simulink model "HighwayLaneFollowingTestBench"  (R2022a)
settings: Solver=ode23tb  StartTime=0.0  StopTime=scenario.StopTime  RelTol=1e-3
PostLoadFcn:
  | helperSLHighwayLaneFollowingSetup
values from neighbouring files (symbols this model uses):
  vehSim3D = repmat(     struct(         'Length', 0,         'RearOverhang', 0,         'InitialPos',[0 0 0],         'InitialRot',[0 0 0]),     numVehicles,1)    [helperSLHighwayLaneFollowingSetup.m]
undefined symbols (not defined in the file or in its folder): assessment, Ts, v_set
libraries: drivingscenarioandsensors x8, sim3dautolib x6, simulink x4, sim3dcameralib x1, sim3dprobsensorlib x1, sim3dlib x1, dspvision x1
CloseFcn:
  | helperSLHighwayLaneFollowingCleanUp
settings Model: SILPILSystemUnderTest=refmodels  Creator=The MathWorks, Inc.  LastModifiedBy=The MathWorks, Inc.
settings SolverCC: AlgebraicLoopSolver=TrustRegion  MaxZcPerStep=1
settings DataIOCC: SaveOutput=off  SaveTime=off  ReturnWorkspaceOutputs=off
settings DebuggingCC: ParameterPrecisionLossMsg=none  UnconnectedInputMsg=warning  UnconnectedOutputMsg=warning  UnconnectedLineMsg=warning  PregeneratedLibrarySubsystemCodeDiagnostic=none  SFMachineParentedDataDiag=warning  ArithmeticOperatorsInVariantConditions=warning
settings HardwareCC: ProdLongLongMode=on
settings SFSimCC: SimUseLocalCustomCode=off
settings RTWCC: RTWUseLocalCustomCode=off  DLArmComputeVersion=19.05
settings GRTTargetCC: RTWCAPISignals=on
settings ConfigComp: CovScope=ReferencedModels  CovIncludeTopModel=off

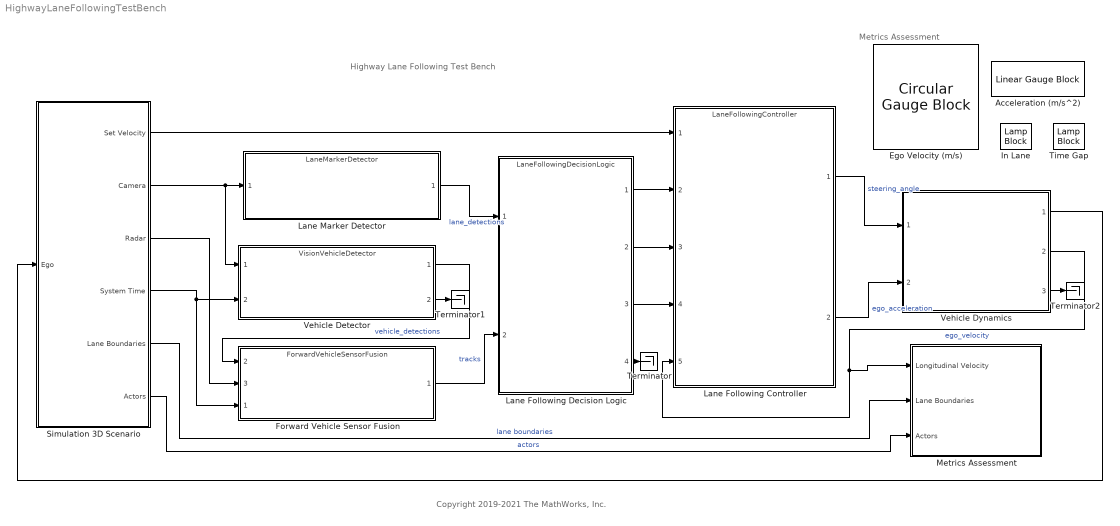
== system HighwayLaneFollowingTestBench ==
  note: Highway Lane Following Test Bench
  note: Metrics Assessment
  note: Copyright 2019-2021 The MathWorks, Inc.
  Acceleration (m/s^2) : LinearGaugeBlock  LabelPosition=Hide  ScaleMin=-6  ScaleMax=6
  Ego Velocity (m/s) : CircularGaugeBlock  LabelPosition=Hide  ScaleMax=50
  Forward Vehicle Sensor Fusion : ModelReference  ModelNameDialog=ForwardVehicleSensorFusion.slx  SimulationMode=Normal  CodeInterface=Top model  ModelReferenceVersion=5.7
      settings: PortSchema="{\"entries\":[{\"content\":{\"sides\":[{\"content\":{\"connectorIds\":[\"In2\",\"In3\",\"In1\"]},\"type\":\"ConnectorPlacement.EquallySpacedRectSide\",\"uuid\":\"7686684e-3ce8-49a8-9c28-78afc562c6cd\"},{\"content\":{\"connectorIds\":[\"Out1\"],\"side\":\"RIGHT\"},\"type\":\"ConnectorPlacement.EquallySpacedRectSide\",\"uuid\":\"c415bca7-2ba8-48d1-9f28-43832dd5ba4e\"},{\"content\":{\"connectorIds\":[],\"side\":\"TOP\"},\"type\":\"ConnectorPlacement.EquallySpacedRectSide\",\"uuid\":\"f22886ed-f0b4-4628-af34-640797a1171b\"}]},\"type\":\"ConnectorPlacement.EquallySpacedConnector\",\"uuid\":\"6b238f4e-3dd4-4f3d-8d3a-ef3e86789fb5\"}],\"packageUris\":[\"http://schema.mathworks.com/mf0/Connector/R2020b\"],\"version\":\"1.0\"}"
  In Lane : LampBlock  LabelPosition=Hide
  Lane Following Controller : ModelReference  ModelNameDialog=LaneFollowingController  SimulationMode=Normal  CodeInterface=Top model  ModelReferenceVersion=5.0
  Lane Following Decision Logic : ModelReference  ModelNameDialog=LaneFollowingDecisionLogic.slx  SimulationMode=Normal  CodeInterface=Top model  ModelReferenceVersion=4.0
  Lane Marker Detector : ModelReference  ModelNameDialog=LaneMarkerDetector.slx  SimulationMode=Normal  CodeInterface=Top model  ModelReferenceVersion=3.0
  Metrics Assessment : Subsystem
  Simulation 3D Scenario : Subsystem  VariantControl=1
  Terminator : Terminator
  Terminator1 : Terminator
  Terminator2 : Terminator
  Time Gap : LampBlock  LabelPosition=Hide
  Vehicle Detector : ModelReference  ModelNameDialog=VisionVehicleDetector.slx  SimulationMode=Normal  CodeInterface=Top model  ModelReferenceVersion=4.0
  Vehicle Dynamics : Subsystem  VariantControl=Variant2  ReferencedSubsystem=BicycleWithForceInput
  wires:
  Vehicle Dynamics/2 -> Lane Following Controller/5, Metrics Assessment/1(Longitudinal Velocity)  "ego_velocity"
  Vehicle Dynamics/1 -> Simulation 3D Scenario/1(Ego)
  Simulation 3D Scenario/6(Actors) -> Metrics Assessment/3(Actors)  "actors"
  Lane Following Controller/1 -> Vehicle Dynamics/1  "steering_angle"
  Lane Following Controller/2 -> Vehicle Dynamics/2  "ego_acceleration"
  Forward Vehicle Sensor Fusion/1 -> Lane Following Decision Logic/2  "tracks"
  Simulation 3D Scenario/5(Lane Boundaries) -> Metrics Assessment/2(Lane Boundaries)  "lane boundaries"
  Simulation 3D Scenario/3(Radar) -> Forward Vehicle Sensor Fusion/3
  Lane Marker Detector/1 -> Lane Following Decision Logic/1  "lane_detections"
  Simulation 3D Scenario/1(Set Velocity) -> Lane Following Controller/1
  Simulation 3D Scenario/4(System Time) -> Forward Vehicle Sensor Fusion/1, Vehicle Detector/2
  Simulation 3D Scenario/2(Camera) -> Vehicle Detector/1, Lane Marker Detector/1
  Lane Following Decision Logic/1 -> Lane Following Controller/2
  Lane Following Decision Logic/2 -> Lane Following Controller/3
  Lane Following Decision Logic/3 -> Lane Following Controller/4
  Vehicle Detector/2 -> Terminator1/1
  Vehicle Detector/1 -> Forward Vehicle Sensor Fusion/2  "vehicle_detections"
  Lane Following Decision Logic/4 -> Terminator/1
  Vehicle Dynamics/3 -> Terminator2/1

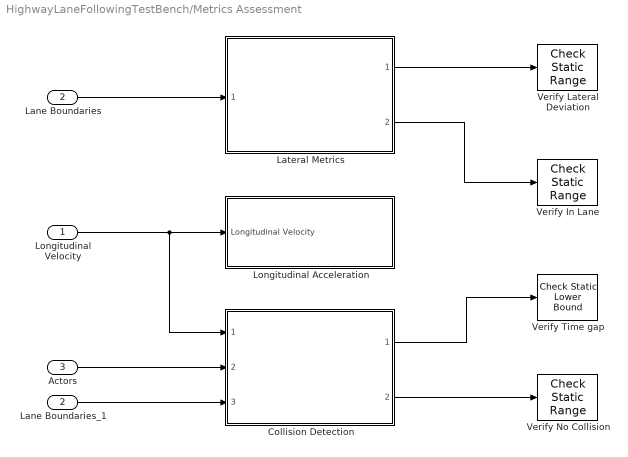
== system HighwayLaneFollowingTestBench/Metrics Assessment ==
  Longitudinal Velocity : Inport
  Lane Boundaries : Inport  Port=2
  Actors : Inport  Port=3
  Collision Detection : Subsystem  ReferencedSubsystem=CollisionDetection
  Lane Boundaries_1 : InportShadow  Port=2
  Lateral Metrics : Subsystem  ReferencedSubsystem=LateralMetrics
  Longitudinal Acceleration : Subsystem
  Verify In Lane : simulink/Model Verification/Check  Static Range  Description=1 <= u <= 1  max=1  max_included=on  min=1  min_included=on  enabled=on  stopWhenAssertionFail=on  export=off  icon=graphic
      settings: SourceProductBaseCode=SL
  Verify Lateral Deviation : simulink/Model Verification/Check  Static Range  Description=-assessment.LateralDeviationMax <= u <= assessment.LateralDeviationMax  max=assessment.LateralDeviationMax  max_included=on  min=-assessment.LateralDeviationMax  min_included=on  enabled=on  stopWhenAssertionFail=on  export=off  icon=graphic
      settings: SourceProductBaseCode=SL
      settings: AttributesFormatString=|
      | ---------------------------------------
      | max = %<max>
      | min = %<min>
  Verify No Collision : simulink/Model Verification/Check  Static Range  Description=0 <= u <= 0  max=0  max_included=on  min=0  min_included=on  enabled=on  stopWhenAssertionFail=on  export=off  icon=graphic
      settings: SourceProductBaseCode=SL
  Verify Time gap : simulink/Model Verification/Check Static  Lower Bound  Description=assessment.TimeGap <= u  min=assessment.TimeGap  min_included=on  enabled=on  stopWhenAssertionFail=on  export=off  icon=graphic
      settings: AttributesFormatString=|
      | ---------------------------------------
      | min = %<min>
  wires:
  Lane Boundaries/1 -> Lateral Metrics/1
  Collision Detection/1 -> Verify Time gap/1
  Lateral Metrics/1 -> Verify Lateral Deviation/1
  Collision Detection/2 -> Verify No Collision/1
  Longitudinal Velocity/1 -> Collision Detection/1, Longitudinal Acceleration/1(Longitudinal Velocity)
  Actors/1 -> Collision Detection/2
  Lateral Metrics/2 -> Verify In Lane/1
  Lane Boundaries_1/1 -> Collision Detection/3

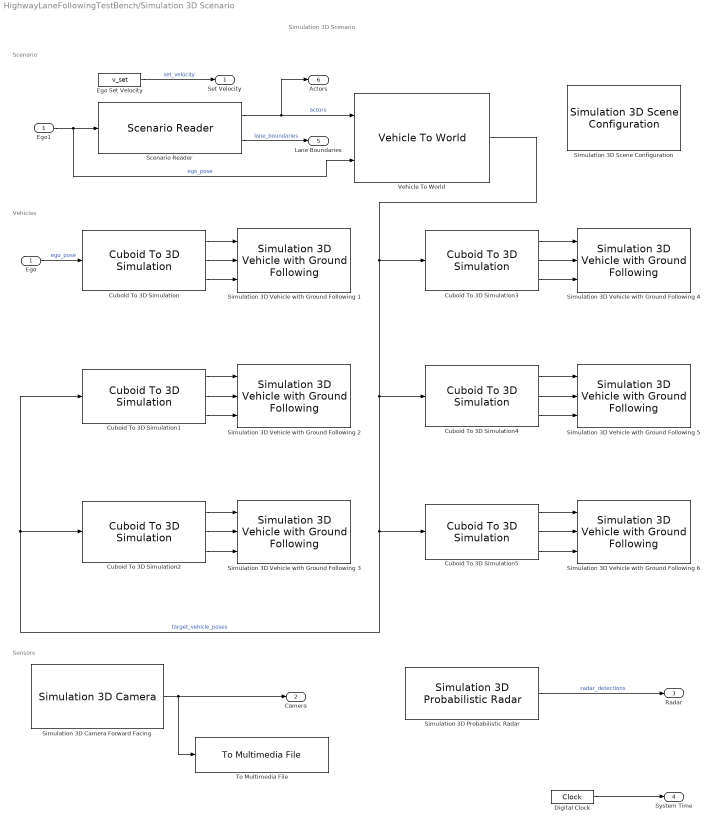
== system HighwayLaneFollowingTestBench/Simulation 3D Scenario ==
  note: Scenario
  note: Vehicles
  note: Simulation 3D Scenario
  note: Sensors
  Ego : Inport
  Cuboid To 3D Simulation : drivingscenarioandsensors/Cuboid To 3D Simulation  SpecifyActorID=off  ActorIDToConvert=1  SimulateUsing=Interpreted execution
      settings: SourceProductBaseCode=DR
  Cuboid To 3D Simulation1 : drivingscenarioandsensors/Cuboid To 3D Simulation  SpecifyActorID=on  ActorIDToConvert=2  SimulateUsing=Interpreted execution
      settings: SourceProductBaseCode=DR
  Cuboid To 3D Simulation2 : drivingscenarioandsensors/Cuboid To 3D Simulation  SpecifyActorID=on  ActorIDToConvert=3  SimulateUsing=Interpreted execution
      settings: SourceProductBaseCode=DR
  Cuboid To 3D Simulation3 : drivingscenarioandsensors/Cuboid To 3D Simulation  SpecifyActorID=on  ActorIDToConvert=4  SimulateUsing=Interpreted execution
      settings: SourceProductBaseCode=DR
  Cuboid To 3D Simulation4 : drivingscenarioandsensors/Cuboid To 3D Simulation  SpecifyActorID=on  ActorIDToConvert=5  SimulateUsing=Interpreted execution
      settings: SourceProductBaseCode=DR
  Cuboid To 3D Simulation5 : drivingscenarioandsensors/Cuboid To 3D Simulation  SpecifyActorID=on  ActorIDToConvert=6  SimulateUsing=Interpreted execution
      settings: SourceProductBaseCode=DR
  Digital Clock : DigitalClock  SampleTime=Ts
  Ego Set Velocity : Constant  Value=v_set  SampleTime=Ts
  Ego1 : InportShadow
  Scenario Reader : drivingscenarioandsensors/Scenario Reader  ScenarioSource=From workspace  ScenarioFileName=dblLaneChangeDrivingScenario.mat  ScenarioVariableName=scenario  OutputCoordinateSystem=Vehicle coordinates  EgoVehicleSource=Input port  EgoVehicleActorID=1  OrientVehiclesOnRoad=off  OutputEgoVehiclePose=off  OutputEgoVehicleState=off  SampleTime=0.1  LaneBoundaryOutput=Ego vehicle lane boundaries  LaneBoundaryDistance=0:0.5:70  LaneBoundaryLocation=Center of lane markings  BusNameSource=Auto  BusName=BusActors  BusNumActorsSource=Scenario  BusNumActors=100  BusName2Source=Auto  BusName2=BusLaneBoundaries  BusNumLaneBoundariesSource=Scenario  BusNumLaneBoundaries=10  BusName3Source=Auto  BusName3=BusEgoActor  BusName4Source=Auto  BusName4=BusEgoState  ShowCoordinateLabels=on  SimulateUsing=Interpreted execution
  Simulation 3D Camera Forward Facing : sim3dcameralib/Simulation 3D Camera  Priority=1  sensorTag=Sim3dSensor1  sensorId=1  sensorName=Sim3dSensor1  vehTagList={'Scene Origin';'SimulinkVehicle1';'SimulinkVehicle4';'SimulinkVehicle5';'SimulinkVehicle6';'vehSim3D(2).InitialRot';'vehSim3D(3).InitialRot'}  vehTag=SimulinkVehicle1  mountLoc=Origin  offsetFlag=on  tmountOffset=camera.PositionSim3d  extTmount=off  rmountOffset=camera.Rotation  extRmount=off  FocalLength=camera.FocalLength  OpticalCenter=camera.PrincipalPoint  ImageSize=camera.ImageSize  RadialDistortion=[0, 0]  TangentialDistortion=[0, 0]  SensorSkew=0  DepthOutportEnabled=off  SemanticOutportEnabled=off  TransformOutportEnabled=off  SampleTime=-1  mountPoint=[0.57 0 1.2]  mountOrientation=[0 0 0]  aMode=3  ID=1
      settings: SourceProductBaseCode=VE,AE,DR,UV,VE
      settings: AttributesFormatString=|
      | -------------------------------------
      | ImageSize = %<ImageSize>
      | OpticalCenter = %<OpticalCenter>
      | FocalLength = %<FocalLength>
      | RadialDistortion = %<RadialDistortion>
      | mountLoc = %<mountLoc>
      | tmountOffset = %<tmountOffset>
      | rmountOffset = %<rmountOffset>
      | Priority = %<Priority>
  Simulation 3D Probabilistic Radar : sim3dprobsensorlib/Simulation 3D Probabilistic Radar  Priority=1  sensorTag=Sim3dSensor2  sensorId=2  sensorName=Sim3dSensor2  vehTagList={'Scene Origin';'SimulinkVehicle1';'SimulinkVehicle4';'SimulinkVehicle5';'SimulinkVehicle6';'vehSim3D(2).InitialRot';'vehSim3D(3).InitialRot'}  vehTag=SimulinkVehicle1  mountLoc=Origin  offsetFlag=on  tmountOffset=radar.PositionSim3d  rmountOffset=radar.Rotation  AzimuthResolution=0.8  ElevationResolution=8  RangeResolution=1  RangeRateResolution=1  AzimuthBiasFraction=0.1  ElevationBiasFraction=0.1  RangeBiasFraction=0.05  RangeRateBiasFraction=0.05  FieldOfView=radar.FieldOfView  DetectionRange=radar.DetectionRanges  RangeRateLimits=[ -100, 100 ]  DetectionProbability=0.9  FalseAlarmRate=1e-6  ReferenceRange=150  ReferenceRCS=0  HasElevation=off  HasRangeRate=on  HasNoise=off  HasFalseAlarms=off  InitialSeedSource=Repeatable  InitialSeed=0  MaxNumDetections=50  DetectionCoordinates=Sensor spherical  SpecifyOutputBusName=off  BusName=BusSimulation3DRadarTruthSensor  SampleTime=-1  mountPoint=[2.424 0 0.8]  mountOrientation=[0 0 0]  aMode=3  ID=2
      settings: SourceProductBaseCode=VE,AE,DR,UV,VE
      settings: AttributesFormatString=|
      | -------------------------------------
      | FieldOfView = %<FieldOfView>
      | AzimuthResolution = %<AzimuthResolution>
      | DetectionCoordinates = %<DetectionCoordinates>
      | mountLoc = %<mountLoc>
      | tmountOffset = %<tmountOffset>
      | rmountOffset = %<rmountOffset>
      | Priority = %<Priority>
  Simulation 3D Scene Configuration : sim3dlib/Simulation 3D Scene Configuration  Priority=0  ProjectFormat=Default Scenes  SceneDesc=Curved road  ProjectName=/mathworks/devel/bat/BR2022ad/build/matlab/toolbox/shared/sim3d_projects/automotive_project/UE4/LinuxNoEditor/AutoVrtlEnv.sh  ScenePath=/Game/Maps/HwStrght  vehTagList={'Scene Origin';'SimulinkVehicle1';'SimulinkVehicle4';'SimulinkVehicle5';'SimulinkVehicle6';'vehSim3D(2).InitialRot';'vehSim3D(3).InitialRot'}  vehTag=SimulinkVehicle1  OpVisEn=off  Ts=0.1  EnableWindow=on  EnableRemoteAccess=off  EnableWeather=off  SunAltitude=40.0  SunAzimuth=90  clouds=10  wind=1  fog=0  rain=0  sensorTag=MainCamera1  sensorId=1  sensorName=MainCamera1  mountLoc=Origin  offsetFlag=off  tmountOffset=[0, 0, 0]  rmountOffset=[0, 0, 0]  HorizontalResolution=1280  VerticalResolution=720  HorizontalFOV=60  mountPoint=[0 0 0]  mountOrientation=[0 0 0]  aMode=3  ID=1
      settings: SourceProductBaseCode=VE,AE,DR,UV,VE
      settings: AttributesFormatString=|
      | -------------------------------------
      | SceneName = %<SceneDesc>
      | Priority = %<Priority>
  Simulation 3D Vehicle with Ground Following 1 : sim3dautolib/Simulation 3D Vehicle with Ground Following  Priority=-1  PassVehMesh=Sedan  MeshPath=/MathWorksSimulation/Vehicles/Muscle/Meshes/SK_MuscleCar.SK_MuscleCar  TrackWidth=1.9  WheelBase=3  WheelRadius=0.35  VehColor=Blue  InitialPos=vehSim3D(1).InitialPos  InitialRot=vehSim3D(1).InitialRot  ActorName=SimulinkVehicle1  SampleTime=-1  ActorType=SimulinkVehicle  ID=1  aMode=3  ActorTag=SimulinkVehicle1  CoordinateScheme=ISO  VehLightsControl=off  HeadlightColor=[ 1, 1, 1 ]  HighBeamIntensity=100000  LowBeamIntensity=60000  HighBeamConeAngle=70  LowBeamConeAngle=70  LeftHeadlightOrientation=[ 0, 0 ]  RightHeadlightOrientation=[ 0, 0 ]  BrakelightIntensity=500  ReverselightIntensity=500  SignallightIntensity=500  SignallightPeriod=1  SignalPulseWidth=50  TransformOutportEnabled=off
      settings: SourceProductBaseCode=VE,AE,DR,UV,VE
      settings: AttributesFormatString=|
      | --------------------------------------
      | ActorName = %<ActorName>
      | PassVehMesh = %<PassVehMesh>
      | VehColor = %<VehColor>
      | InitialPos = %<InitialPos>
      | InitialRot = %<InitialRot>
      | Priority = %<Priority>
  Simulation 3D Vehicle with Ground Following 2 : sim3dautolib/Simulation 3D Vehicle with Ground Following  Priority=-1  PassVehMesh=Sedan  MeshPath=/MathWorksSimulation/Vehicles/Muscle/Meshes/SK_MuscleCar.SK_MuscleCar  TrackWidth=1.9  WheelBase=3  WheelRadius=0.35  VehColor=Red  InitialPos=vehSim3D(2).InitialPos  InitialRot=vehSim3D(2).InitialRot  ActorName=vehSim3D(2).InitialRot  SampleTime=-1  ActorType=SimulinkVehicle  ID=C  aMode=3  ActorTag=vehSim3D(2).InitialRot  CoordinateScheme=ISO  VehLightsControl=off  HeadlightColor=[ 1, 1, 1 ]  HighBeamIntensity=100000  LowBeamIntensity=60000  HighBeamConeAngle=70  LowBeamConeAngle=70  LeftHeadlightOrientation=[ 0, 0 ]  RightHeadlightOrientation=[ 0, 0 ]  BrakelightIntensity=500  ReverselightIntensity=500  SignallightIntensity=500  SignallightPeriod=1  SignalPulseWidth=50  TransformOutportEnabled=off
      settings: SourceProductBaseCode=VE,AE,DR,UV,VE
      settings: AttributesFormatString=|
      | --------------------------------------
      | ActorName = %<ActorName>
      | PassVehMesh = %<PassVehMesh>
      | VehColor = %<VehColor>
      | InitialPos = %<InitialPos>
      | InitialRot = %<InitialRot>
      | Priority = %<Priority>
  Simulation 3D Vehicle with Ground Following 3 : sim3dautolib/Simulation 3D Vehicle with Ground Following  Priority=-1  PassVehMesh=Muscle car  MeshPath=/MathWorksSimulation/Vehicles/Muscle/Meshes/SK_MuscleCar.SK_MuscleCar  TrackWidth=1.9  WheelBase=3  WheelRadius=0.35  VehColor=Black  InitialPos=vehSim3D(3).InitialPos  InitialRot=vehSim3D(3).InitialRot  ActorName=vehSim3D(3).InitialRot  SampleTime=-1  ActorType=SimulinkVehicle  ID=C  aMode=3  ActorTag=vehSim3D(3).InitialRot  CoordinateScheme=ISO  VehLightsControl=off  HeadlightColor=[ 1, 1, 1 ]  HighBeamIntensity=100000  LowBeamIntensity=60000  HighBeamConeAngle=70  LowBeamConeAngle=70  LeftHeadlightOrientation=[ 0, 0 ]  RightHeadlightOrientation=[ 0, 0 ]  BrakelightIntensity=500  ReverselightIntensity=500  SignallightIntensity=500  SignallightPeriod=1  SignalPulseWidth=50  TransformOutportEnabled=off
      settings: SourceProductBaseCode=VE,AE,DR,UV,VE
      settings: AttributesFormatString=|
      | --------------------------------------
      | ActorName = %<ActorName>
      | PassVehMesh = %<PassVehMesh>
      | VehColor = %<VehColor>
      | InitialPos = %<InitialPos>
      | InitialRot = %<InitialRot>
      | Priority = %<Priority>
  Simulation 3D Vehicle with Ground Following 4 : sim3dautolib/Simulation 3D Vehicle with Ground Following  Priority=-1  PassVehMesh=Hatchback  MeshPath=/MathWorksSimulation/Vehicles/Muscle/Meshes/SK_MuscleCar.SK_MuscleCar  TrackWidth=1.9  WheelBase=3  WheelRadius=0.35  VehColor=Orange  InitialPos=vehSim3D(4).InitialPos  InitialRot=vehSim3D(4).InitialRot  ActorName=SimulinkVehicle4  SampleTime=-1  ActorType=SimulinkVehicle  ID=4  aMode=3  ActorTag=SimulinkVehicle4  CoordinateScheme=ISO  VehLightsControl=off  HeadlightColor=[ 1, 1, 1 ]  HighBeamIntensity=100000  LowBeamIntensity=60000  HighBeamConeAngle=70  LowBeamConeAngle=70  LeftHeadlightOrientation=[ 0, 0 ]  RightHeadlightOrientation=[ 0, 0 ]  BrakelightIntensity=500  ReverselightIntensity=500  SignallightIntensity=500  SignallightPeriod=1  SignalPulseWidth=50  TransformOutportEnabled=off
      settings: SourceProductBaseCode=VE,AE,DR,UV,VE
      settings: AttributesFormatString=|
      | --------------------------------------
      | ActorName = %<ActorName>
      | PassVehMesh = %<PassVehMesh>
      | VehColor = %<VehColor>
      | InitialPos = %<InitialPos>
      | InitialRot = %<InitialRot>
      | Priority = %<Priority>
  Simulation 3D Vehicle with Ground Following 5 : sim3dautolib/Simulation 3D Vehicle with Ground Following  Priority=-1  PassVehMesh=Small pickup truck  MeshPath=/MathWorksSimulation/Vehicles/Muscle/Meshes/SK_MuscleCar.SK_MuscleCar  TrackWidth=1.9  WheelBase=3  WheelRadius=0.35  VehColor=Green  InitialPos=vehSim3D(5).InitialPos  InitialRot=vehSim3D(5).InitialRot  ActorName=SimulinkVehicle5  SampleTime=-1  ActorType=SimulinkVehicle  ID=5  aMode=3  ActorTag=SimulinkVehicle5  CoordinateScheme=ISO  VehLightsControl=off  HeadlightColor=[ 1, 1, 1 ]  HighBeamIntensity=100000  LowBeamIntensity=60000  HighBeamConeAngle=70  LowBeamConeAngle=70  LeftHeadlightOrientation=[ 0, 0 ]  RightHeadlightOrientation=[ 0, 0 ]  BrakelightIntensity=500  ReverselightIntensity=500  SignallightIntensity=500  SignallightPeriod=1  SignalPulseWidth=50  TransformOutportEnabled=off
      settings: SourceProductBaseCode=VE,AE,DR,UV,VE
      settings: AttributesFormatString=|
      | --------------------------------------
      | ActorName = %<ActorName>
      | PassVehMesh = %<PassVehMesh>
      | VehColor = %<VehColor>
      | InitialPos = %<InitialPos>
      | InitialRot = %<InitialRot>
      | Priority = %<Priority>
  Simulation 3D Vehicle with Ground Following 6 : sim3dautolib/Simulation 3D Vehicle with Ground Following  Priority=-1  PassVehMesh=Sport utility vehicle  MeshPath=/MathWorksSimulation/Vehicles/Muscle/Meshes/SK_MuscleCar.SK_MuscleCar  TrackWidth=1.9  WheelBase=3  WheelRadius=0.35  VehColor=Blue  InitialPos=vehSim3D(6).InitialPos  InitialRot=vehSim3D(6).InitialRot  ActorName=SimulinkVehicle6  SampleTime=-1  ActorType=SimulinkVehicle  ID=6  aMode=3  ActorTag=SimulinkVehicle6  CoordinateScheme=ISO  VehLightsControl=off  HeadlightColor=[ 1, 1, 1 ]  HighBeamIntensity=100000  LowBeamIntensity=60000  HighBeamConeAngle=70  LowBeamConeAngle=70  LeftHeadlightOrientation=[ 0, 0 ]  RightHeadlightOrientation=[ 0, 0 ]  BrakelightIntensity=500  ReverselightIntensity=500  SignallightIntensity=500  SignallightPeriod=1  SignalPulseWidth=50  TransformOutportEnabled=off
      settings: SourceProductBaseCode=VE,AE,DR,UV,VE
      settings: AttributesFormatString=|
      | --------------------------------------
      | ActorName = %<ActorName>
      | PassVehMesh = %<PassVehMesh>
      | VehColor = %<VehColor>
      | InitialPos = %<InitialPos>
      | InitialRot = %<InitialRot>
      | Priority = %<Priority>
  To Multimedia File : dspvision/To Multimedia File  outputFilename=forwardFacingCamera.mp4  streamSelection=Video only  videoCompressor=None (uncompressed)  audioCompressor=None (uncompressed)  imagePorts=One multidimensional signal  fileType=MPEG4  audioDatatype=Determine from input data type  fourcc=RGB  videoQuality=75  mj2000CompFactor=10
  Vehicle To World : drivingscenarioandsensors/Vehicle To World  BusNameSource=Auto  BusName=BusVehicleToWorldActors  SimulateUsing=Interpreted execution
      settings: SourceProductBaseCode=DR
  Set Velocity : Outport  Unit=m/s  VectorParamsAs1DForOutWhenUnconnected=off
  Camera : Outport  Port=2  VectorParamsAs1DForOutWhenUnconnected=off
  Radar : Outport  Port=3  VectorParamsAs1DForOutWhenUnconnected=off
  System Time : Outport  Port=4  VectorParamsAs1DForOutWhenUnconnected=off
  Lane Boundaries : Outport  Port=5
  Actors : Outport  Port=6
  wires:
  Digital Clock/1 -> System Time/1
  Cuboid To 3D Simulation/2 -> Simulation 3D Vehicle with Ground Following 1/2
  Cuboid To 3D Simulation/1 -> Simulation 3D Vehicle with Ground Following 1/1
  Cuboid To 3D Simulation/3 -> Simulation 3D Vehicle with Ground Following 1/3
  Ego/1 -> Cuboid To 3D Simulation/1  "ego_pose"
  Cuboid To 3D Simulation1/2 -> Simulation 3D Vehicle with Ground Following 2/2
  Cuboid To 3D Simulation1/1 -> Simulation 3D Vehicle with Ground Following 2/1
  Cuboid To 3D Simulation1/3 -> Simulation 3D Vehicle with Ground Following 2/3
  Simulation 3D Probabilistic Radar/1 -> Radar/1  "radar_detections"
  Simulation 3D Camera Forward Facing/1 -> Camera/1, To Multimedia File/1
  Scenario Reader/1 -> Vehicle To World/1, Actors/1  "actors"
  Vehicle To World/1 -> Cuboid To 3D Simulation3/1, Cuboid To 3D Simulation4/1, Cuboid To 3D Simulation2/1, Cuboid To 3D Simulation1/1, Cuboid To 3D Simulation5/1  "target_vehicle_poses"
  Cuboid To 3D Simulation3/2 -> Simulation 3D Vehicle with Ground Following 4/2
  Cuboid To 3D Simulation3/3 -> Simulation 3D Vehicle with Ground Following 4/3
  Cuboid To 3D Simulation2/2 -> Simulation 3D Vehicle with Ground Following 3/2
  Cuboid To 3D Simulation3/1 -> Simulation 3D Vehicle with Ground Following 4/1
  Cuboid To 3D Simulation2/3 -> Simulation 3D Vehicle with Ground Following 3/3
  Cuboid To 3D Simulation2/1 -> Simulation 3D Vehicle with Ground Following 3/1
  Cuboid To 3D Simulation4/3 -> Simulation 3D Vehicle with Ground Following 5/3
  Cuboid To 3D Simulation5/2 -> Simulation 3D Vehicle with Ground Following 6/2
  Cuboid To 3D Simulation5/3 -> Simulation 3D Vehicle with Ground Following 6/3
  Cuboid To 3D Simulation5/1 -> Simulation 3D Vehicle with Ground Following 6/1
  Cuboid To 3D Simulation4/2 -> Simulation 3D Vehicle with Ground Following 5/2
  Cuboid To 3D Simulation4/1 -> Simulation 3D Vehicle with Ground Following 5/1
  Scenario Reader/2 -> Lane Boundaries/1  "lane_boundaries"
  Ego1/1 -> Vehicle To World/2, Scenario Reader/1  "ego_pose"
  Ego Set Velocity/1 -> Set Velocity/1  "set_velocity"

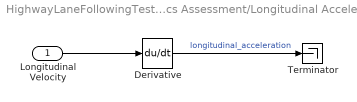
== system HighwayLaneFollowingTestBench/Metrics Assessment/Longitudinal Acceleration ==
  Longitudinal Velocity : Inport
  Derivative : Derivative
  Terminator : Terminator
  wires:
  Derivative/1 -> Terminator/1  "longitudinal_acceleration"
  Longitudinal Velocity/1 -> Derivative/1
